simulink model "rpi_camera_feed"  (R2022b)
settings: Solver=FixedStepDiscrete  StartTime=0.0  StopTime=8  RelTol=1e-3  EnableMultiTasking=on
values from neighbouring files (symbols this model uses):
  A = [1.06559801427  0.0478097134081  -0.0142426631232; 0.0478097134081  0.959164863261  -0.0359507847494; -0.0142426631232  -0.0359507847494  0.982079248423]    [mag_cal.mat]
  b = [2.14306210308 15.720848335 -0.863601368467]    [mag_cal.mat]
undefined symbols (not defined in the file or in its folder): image_strip_thresh, image_strip_thresh_abs
libraries: raspberrypiIMUsensorslib x1, dspsigops x1, raspberrypiAVlib x1
settings Model: Creator=sjohnson  LastModifiedBy=sjohnson
settings SolverCC: PositivePriorityOrder=on
settings OptimizationCC: EnhancedBackFolding=on  PassReuseOutputArgsAs=Individual arguments  ZeroExternalMemoryAtStartup=off  ZeroInternalMemoryAtStartup=off  MaxStackSize=64  OptimizeBlockOrder=speed  DifferentSizesBufferReuse=on  OptimizationCustomize=off  EfficientTunableParamExpr=on
settings DebuggingCC: ParameterTunabilityLossMsg=error
settings HardwareCC: ProdBitPerPointer=32  ProdBitPerSizeT=32  ProdBitPerPtrDiffT=32  ProdLargestAtomicInteger=Long  ProdLargestAtomicFloat=Double  ProdWordSize=32  ProdLongLongMode=on  ProdHWDeviceType=ARM Compatible->ARM Cortex  UseEmbeddedCoderFeatures=off  UseSimulinkCoderFeatures=off
settings RTWCC: Description=Embedded Coder  SystemTargetFile=ert.tlc  HardwareBoard=Raspberry Pi  TLCOptions="-aInlineSetEventsForThisBaseRateFcn=TLC_FALSE -aSuppressMultiTaskScheduler=TLC_FALSE  -aRateBasedStepFcn=0"  TemplateMakefile=ert_default_tmf  Toolchain=GNU GCC Embedded Linux  BuildConfiguration=Faster Runs
settings CodeAppCC: ForceParamTrailComments=on  IgnoreCustomStorageClasses=off  OperatorAnnotations=on  SimulinkDataObjDesc=on  SFDataObjDesc=on  MangleLength=10  InsertBlockDesc=on
settings ERTTargetCC: SupportNonInlinedSFcns=on  SupportVariableSizeSignals=on  ExtModeTransport=2  ExtModeStaticAlloc=on  ExtModeMexFile=ext_xcp  ExtModeIntrfLevel=Level2 - Open

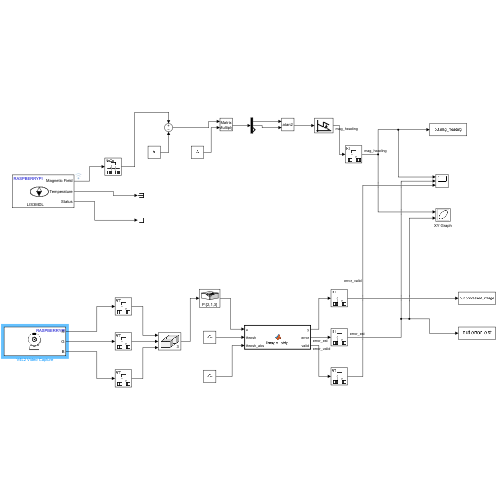
[thumbnail: Simulink's stored preview of the top-level diagram]
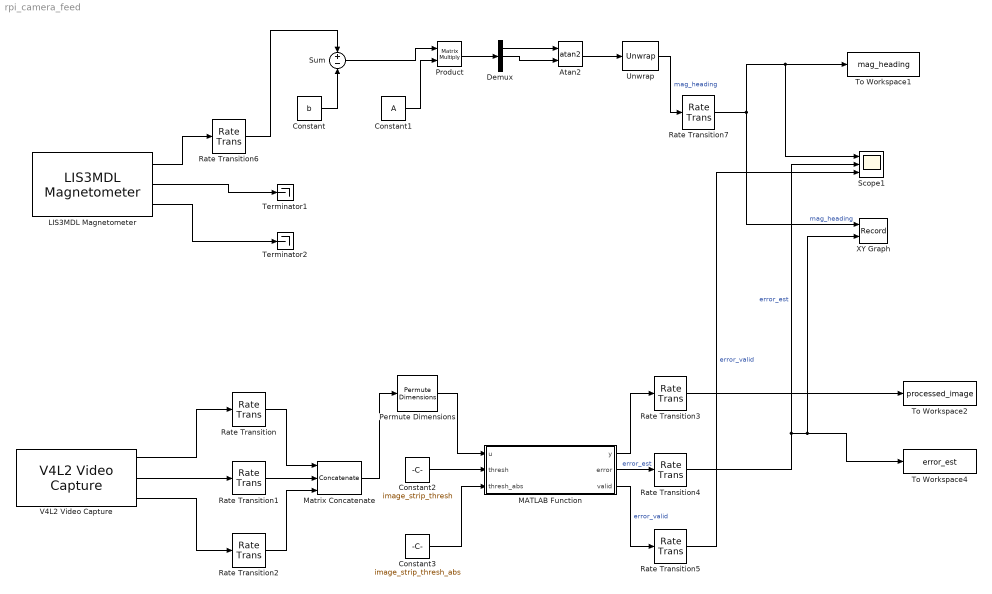
== system rpi_camera_feed ==
  Atan2 : Trigonometry  Operator=atan2
  Constant : Constant  Value=b
  Constant1 : Constant  Value=A
  Constant2 : Constant  Value=image_strip_thresh
  Constant3 : Constant  Value=image_strip_thresh_abs
  Demux : Demux  Outputs=3
  LIS3MDL Magnetometer : raspberrypiIMUsensorslib/LIS3MDL Magnetometer  I2CModule=1  I2CAddress=0x1E  IsActiveMagnetometer=on  IsActiveTemperature=on  IsStatus=on  SampleTime=-1  MagnetometerRange=+/- 400 uT  MagnetometerODR=40 Hz
  MATLAB Function : MATLAB Function  TreatAsAtomicUnit=on
  Matrix Concatenate : Concatenate  NumInputs=3  Mode=Multidimensional array  ConcatenateDimension=3
  Permute Dimensions : PermuteDimensions  Order=[2,1,3]
  Product : Product  Multiplication=Matrix(*)
  Rate Transition{,1..7} (8 alike) : RateTransition
  Scope1 : Scope  NumInputPorts=3
  Sum : Sum  Inputs=+-
  Terminator1 : Terminator
  Terminator2 : Terminator
  To Workspace1 : ToWorkspace  VariableName=mag_heading  SaveFormat=Structure With Time  SampleTime=-1
  To Workspace2 : ToWorkspace  VariableName=processed_image  SaveFormat=Structure With Time  SampleTime=-1
  To Workspace4 : ToWorkspace  VariableName=error_est  SaveFormat=Structure With Time  SampleTime=-1
  Unwrap : dspsigops/Unwrap  tol=pi  InputProcessing=Columns as channels (frame based)  running=off
  V4L2 Video Capture : raspberrypiAVlib/V4L2 Video Capture  DeviceName=/dev/video0  Resolution=640x480  CustomResolution=[ 1024, 768 ]  PixelFormat=RGB  SampleTime=0.03  pixelOrder=planar  simOutput=Colorbars  imSizeSelection=320x240  imSize=[640, 480]  roi=[0, 0, 640, 480]  m_devName='/dev/video0'  blockPlatform=LINUX  HorizontalFlip=off  VerticalFlip=off  Brightness=0.5  Saturation=0.5  Contrast=0.5  Sharpness=0.5  CameraPan=0  CameraTilt=0  CameraZoom=0.5  EnableManualFocus=off  ManualFocus=0.5
  XY Graph : Record  FileSettingsInternal="{\"entries\":[{\"content\":{\"excelSettings\":{\"content\":{},\"type\":\"Streamout.ExcelSettings\"}},\"type\":\"Streamout.FileSettingStorage\",\"uuid\":\"2b484738-ae2a-40cb-a55f-07fc6213caa6\"}],\"packageUris\":[\"http://schema.mathworks.com/mf0/streamout_blocks/R2020a\"],\"version\":\"1.0\"}"  Layout=[1 1]  SignalsInternal="{\"entries\":[{\"content\":{\"signals\":[{\"content\":{\"blockPath\":[\"rpi_camera_feed/XY Graph\"],\"channel\":[],\"dimensions\":[1],\"domain\":\"rpi_camera_feed/XY Graph\",\"lineColor\":\"#139fff\",\"plots\":[1],\"port\":2,\"sid\":[\"35\"],\"signalID\":85515,\"signalName\":\"error_est\"},\"type\":\"RecordBlkView.Signal\",\"uuid\":\"8c927ccb-9d47-450b-aa73-6345e4008edb\"},{\"content\":{\"blockPath\":[\"rpi_camera_feed/XY Graph\"],\"channel\":[],\"dimensions\":[1,1],\"domain\":\"rpi_camera_feed/XY Graph\",\"lineColor\":\"#a2142f\",\"plots\":[1],\"port\":1,\"sid\":[\"35\"],\"signalID\":85523,\"signalName\":\"mag_heading\"},\"type\":\"RecordBlkView.Signal\",\"uuid\":\"759338ac-61df-4106-8891-b7dd5056d659\"}]},\"type\":\"RecordBlkView.InputSignals\",\"uuid\":\"f6128c08-35a4-4412-8a20-4a5de038ac7d\"}],\"packageUris\":[\"http://schema.mathworks.com/mf0/streamout_blocks/R2020a\"],\"version\":\"1.0\"}"  VisualizationBindings="{\"xyplotplugin\":{\"info\":[{\"series\":[{\"bindingParametersList\":[{\"parameter\":\"X-Axis\",\"signalID\":85523,\"signalName\":\"mag_heading\"},{\"parameter\":\"Y-Axis\",\"signalID\":85515,\"signalName\":\"error_est\"}],\"seriesID\":15936}],\"subplotID\":1}]}}"  CompatibilityTag=XY
  wires:
  V4L2 Video Capture/1 -> Rate Transition/1
  V4L2 Video Capture/2 -> Rate Transition1/1
  V4L2 Video Capture/3 -> Rate Transition2/1
  Permute Dimensions/1 -> MATLAB Function/1(u)
  Demux/1 -> Atan2/1
  Atan2/1 -> Unwrap/1
  Constant/1 -> Sum/2
  Demux/2 -> Atan2/2
  Sum/1 -> Product/1
  Product/1 -> Demux/1
  Rate Transition6/1 -> Sum/1
  Constant1/1 -> Product/2
  Constant2/1 -> MATLAB Function/2(thresh)
  Rate Transition3/1 -> To Workspace2/1
  Matrix Concatenate/1 -> Permute Dimensions/1
  LIS3MDL Magnetometer/2 -> Terminator1/1
  LIS3MDL Magnetometer/3 -> Terminator2/1
  Rate Transition7/1 -> Scope1/1, To Workspace1/1, XY Graph/1  "mag_heading"
  Rate Transition4/1 -> Scope1/2, XY Graph/2, To Workspace4/1  "error_est"
  Rate Transition5/1 -> Scope1/3  "error_valid"
  Constant3/1 -> MATLAB Function/3(thresh_abs)
  Rate Transition/1 -> Matrix Concatenate/1
  Rate Transition1/1 -> Matrix Concatenate/2
  Rate Transition2/1 -> Matrix Concatenate/3
  MATLAB Function/1(y) -> Rate Transition3/1
  MATLAB Function/2(error) -> Rate Transition4/1  "error_est"
  MATLAB Function/3(valid) -> Rate Transition5/1  "error_valid"
  LIS3MDL Magnetometer/1 -> Rate Transition6/1
  Unwrap/1 -> Rate Transition7/1  "mag_heading"

== matlab function rpi_camera_feed/MATLAB Function ==
  data: u input; y output; error output; valid output; thresh input; thresh_abs input
function [y, error, valid] = image_strip(u, thresh, thresh_abs)
% trim out horizontal slice of image
y = u(325:425, :, :);
dy = double(y);
redness = dy(:,:,1)./vecnorm(dy,1,3) .* dy(:,:,1)>thresh_abs;
y_reduction = max(redness,[],1);
fmin = find(y_reduction>thresh, 1, 'first');
fmax = find(y_reduction>thresh, 1, 'last');
if isempty(fmin) | isempty(fmax)
    valid = 0;
    error = nan;
else
    valid = 1;
    min_value = [find(y_reduction>thresh, 1, 'first')];
    max_value = [find(y_reduction>thresh, 1, 'last')];
    error = ((max_value(1) + min_value(1))/2 - 320)/320;
end
